simulink model "ex_han2_2017a"  (Simulink 8.9)
settings: Solver=FixedStepAuto  StartTime=0.0  StopTime=10  FixedStep=0.001  RelTol=1e-3
undefined symbols (not defined in the file or in its folder): aa, b, bet, bet1, d, h, r, T
settings Model: SuppressorTable=22 serialization::archive 11 0 6 0 0 0 11 0  Creator=Arthur  LastModifiedBy=rastronaut
settings DataIOCC: LimitDataPoints=off  SaveFormat=Dataset  SignalLoggingSaveFormat=Dataset
settings OptimizationCC: LifeSpan=auto
settings DebuggingCC: UnderspecifiedInitializationDetection=Simplified  MergeDetectMultiDrivingBlocksExec=error  FcnCallInpInsideContextMsg=error  StateNameClashWarn=none  SFUnexpectedBacktrackingDiag=error  SFNoUnconditionalDefaultTransitionDiag=error  SFExecutionAtInitializationDiag=warning
settings HardwareCC: ProdBitPerPointer=64  ProdBitPerSizeT=64  ProdBitPerPtrDiffT=64  ProdLargestAtomicFloat=Float  ProdIntDivRoundTo=Zero  ProdEndianess=LittleEndian  ProdWordSize=64  ProdHWDeviceType=Intel->x86-64 (Windows64)
settings ModelReferenceCC: PropagateSignalLabelsOutOfModel=on
settings GRTTargetCC: TargetLangStandard=C99 (ISO)  GeneratePreprocessorConditionals=Use local settings  CombineOutputUpdateFcns=on  GRTInterface=off
settings ConfigComp: CovMetricSettings=dwe  CovHtmlReporting=off  CovSaveCumulativeToWorkspaceVar=off  CovSaveSingleToWorkspaceVar=off  CovExternalEMLEnable=on

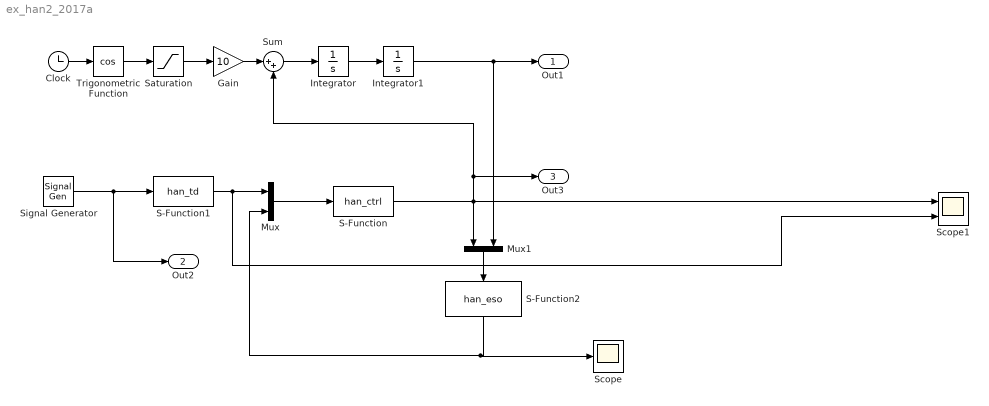
== system ex_han2_2017a ==
  Clock : Clock
  Gain : Gain  Gain=10
  Integrator : Integrator
  Integrator1 : Integrator
  Mux : Mux  Inputs=2
  Mux1 : Mux  Inputs=2
  S-Function : S-Function  FunctionName=han_ctrl  Parameters=aa,bet1,b,d  SFunctionDeploymentMode=off  EnableBusSupport=off
  S-Function1 : S-Function  FunctionName=han_td  Parameters=r,h,T  SFunctionDeploymentMode=off  EnableBusSupport=off
  S-Function2 : S-Function  FunctionName=han_eso  Parameters=d,bet,b,T  SFunctionDeploymentMode=off  EnableBusSupport=off
  Saturation : Saturate
  Scope : Scope
  Scope1 : Scope  NumInputPorts=2
  Signal Generator : SignalGenerator  WaveForm=square  Frequency=0.1
  Sum : Sum  Inputs=|++
  Trigonometric Function : Trigonometry  Operator=cos
  Out1 : Outport  SignalName=Saída
  Out2 : Outport  Port=2  SignalName=Entrada
  Out3 : Outport  Port=3  SignalName=Controle
  wires:
  Mux/1 -> S-Function/1
  Integrator1/1 -> Mux1/2, Out1/1
  Integrator/1 -> Integrator1/1
  Sum/1 -> Integrator/1
  Trigonometric Function/1 -> Saturation/1
  Clock/1 -> Trigonometric Function/1
  Signal Generator/1 -> Out2/1, S-Function1/1
  S-Function/1 -> Scope1/1, Mux1/1, Out3/1, Sum/2
  Mux1/1 -> S-Function2/1
  Saturation/1 -> Gain/1
  Gain/1 -> Sum/1
  S-Function2/1 -> Scope/1, Mux/2
  S-Function1/1 -> Scope1/2, Mux/1
